simulink model "rlBallandPlate"  (R2023a)
settings: Solver=ode45  StartTime=0.0  StopTime=40  RelTol=1e-3
undefined symbols (not defined in the file): DiscIntNeverNeededParam, Ts
libraries: simulink x3, rllib x1
settings Model: Creator=The MathWorks, Inc.  LastModifiedBy=danieludekwe
settings SolverCC: AlgebraicLoopSolver=TrustRegion  MaxZcPerStep=1
settings DataIOCC: DSMLogging=off  ReturnWorkspaceOutputs=off
settings OptimizationCC: ReuseModelBlockBuffer=off
settings DebuggingCC: UnconnectedInputMsg=warning  UnconnectedOutputMsg=warning  UnconnectedLineMsg=warning
settings HardwareCC: ProdBitPerLong=64  ProdHWDeviceType=Apple->ARM64
settings ModelReferenceCC: EnableRefExpFcnMdlSchedulingChecks=on
settings RTWCC: DLArmComputeVersion=19.05
settings ExplorerConfigSet: InternalSimMechanicsExplorerSettings="<ExplorerConfiguration><canonicalview>default</canonicalview><AnimationSetting><BasePlaybackSpeed>1.0</BasePlaybackSpeed><PlaybackSpeedFactor>1.0</PlaybackSpeedFactor></AnimationSetting><TilePanel><TileInfo><Tiles Columns=\"1\" Count=\"1\" Rows=\"1\"><Column Weight=\"1\"/><Row Weight=\"1\"/><Tile Height=\"1\" Width=\"1\" X=\"0\" Y=\"0\"/></Tiles></TileInfo><SceneInfo><SceneViewer><BGColor><R>1</R><G>1</G><B>1</B></BGColor><Camera><DoPerspective>off</DoPerspective><Position><X>0.835449044511457073</X><Y>-0.495506913595096854</Y><Z>0.970261214764596258</Z></Position><Center><X>0.258098775321831175</X><Y>0.0818433555945289881</Y><Z>0.392910945574970416</Z></Center><Up><X>-0.408248290463863073</X><Y>0.408248290463863073</Y><Z>0.816496580927726145</Z></Up><ViewLimDist>1</ViewLimDist><YLim>0.340419242978096004</YLim><XLim>0.488995507299471222</XLim></Camera></SceneViewer></SceneInfo></TilePanel><MechEditorPanel><Cameras/><GfxPanelCameraMap/><VideoCreator><PlaybackSpeedRatio>1.0</PlaybackSpeedRatio><FrameRate>30</FrameRate><VideoFormat>Motion JPEG AVI</VideoFormat><FrameSize>auto</FrameSize></VideoCreator></MechEditorPanel></ExplorerConfiguration>"

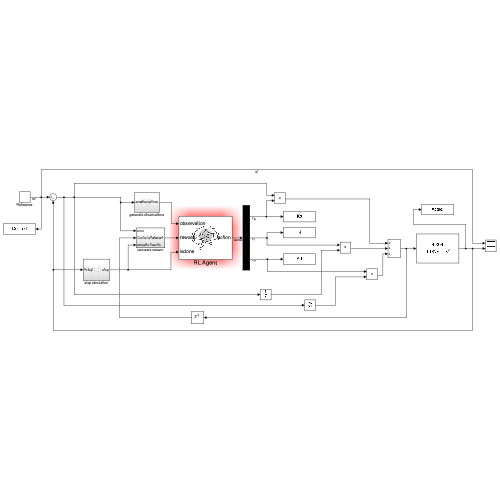
[thumbnail: Simulink's stored preview of the top-level diagram]
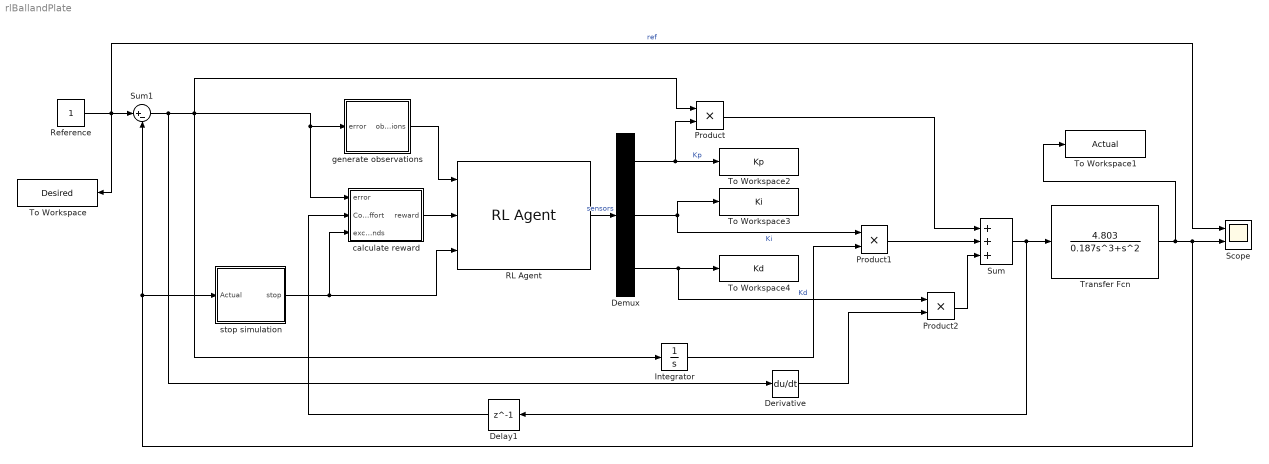
== system rlBallandPlate ==
  Delay1 : Delay  DelayLength=1
  Demux : Demux  Outputs=3
  Derivative : Derivative  CoefficientInTFapproximation=0
  Integrator : Integrator
  Product : Product
  Product1 : Product
  Product2 : Product
  RL Agent : rllib/RL Agent  Agent=agent  ExternalActionAsInput=off  ProvideLastAction=off  ProvideCumRwd=off  TreatAsDirectFeedthrough=on  UseStrictObservationDataTypes=off
  Reference : Constant
  Scope : Scope  NumInputPorts=2
  Sum : Sum  Inputs=+++
  Sum1 : Sum  Inputs=|+-  SaturateOnIntegerOverflow=on
  To Workspace : ToWorkspace  VariableName=Desired  SampleTime=-1
  To Workspace1 : ToWorkspace  VariableName=Actual  SampleTime=-1
  To Workspace2 : ToWorkspace  VariableName=Kp  SaveFormat=Structure With Time  SampleTime=-1
  To Workspace3 : ToWorkspace  VariableName=Ki  SaveFormat=Structure With Time  SampleTime=-1
  To Workspace4 : ToWorkspace  VariableName=Kd  SaveFormat=Structure With Time  SampleTime=-1
  Transfer Fcn : TransferFcn  Numerator=4.803  Denominator=[0.187 1 0 0]
  calculate reward : Subsystem
  generate observations : Subsystem
  stop simulation : Subsystem
  wires:
  generate observations/1(observations) -> RL Agent/1
  stop simulation/1(stop) -> RL Agent/3, calculate reward/3(exceeds bounds)
  Transfer Fcn/1 -> To Workspace1/1, Scope/2, stop simulation/1(Actual), Sum1/2
  RL Agent/1 -> Demux/1  "sensors"
  Reference/1 -> To Workspace/1, Sum1/1, Scope/1  "ref"
  Sum1/1 -> calculate reward/1(error), generate observations/1(error), Integrator/1, Product/1, Derivative/1
  Delay1/1 -> calculate reward/2(Control effort)
  calculate reward/1(reward) -> RL Agent/2
  Demux/2 -> To Workspace3/1, Product1/1  "Ki"
  Demux/3 -> To Workspace4/1, Product2/1  "Kd"
  Product1/1 -> Sum/2
  Product/1 -> Sum/1
  Product2/1 -> Sum/3
  Sum/1 -> Delay1/1, Transfer Fcn/1
  Derivative/1 -> Product2/2
  Integrator/1 -> Product1/2
  Demux/1 -> To Workspace2/1, Product/2  "Kp"

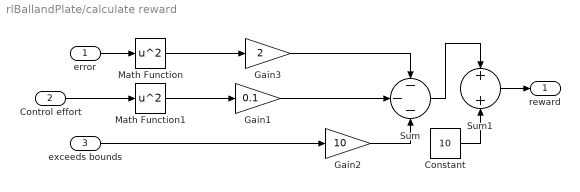
== system rlBallandPlate/calculate reward ==
  error : Inport
  Control effort : Inport  Port=2
  exceeds bounds : Inport  Port=3
  Constant : Constant  Value=10
  Gain1 : Gain  Gain=0.1
  Gain2 : Gain  Gain=10
  Gain3 : Gain  Gain=2
  Math Function : Math  Operator=square
  Math Function1 : Math  Operator=square
  Sum : Sum  Inputs=---  OutDataTypeStr=double
  Sum1 : Sum  OutDataTypeStr=double
  reward : Outport  VectorParamsAs1DForOutWhenUnconnected=off
  wires:
  exceeds bounds/1 -> Gain2/1
  error/1 -> Math Function/1
  Math Function/1 -> Gain3/1
  Gain3/1 -> Sum/1
  Sum/1 -> Sum1/1
  Constant/1 -> Sum1/2
  Sum1/1 -> reward/1
  Math Function1/1 -> Gain1/1
  Gain2/1 -> Sum/3
  Control effort/1 -> Math Function1/1
  Gain1/1 -> Sum/2

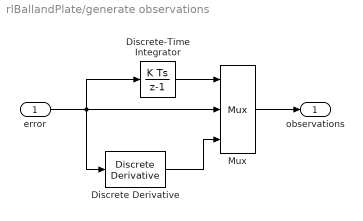
== system rlBallandPlate/generate observations ==
  error : Inport
  Discrete Derivative : simulink/Discrete/Discrete Derivative  gainval=1.0  ICPrevScaledInput=0.0  OutMin=[]  OutMax=[]  OutDataType=fixdt(1, 16)  OutScaling=2^-10  DoSatur=off
  Discrete-Time Integrator : DiscreteIntegrator  SampleTime=Ts  ICPrevOutput=DiscIntNeverNeededParam  ICPrevScaledInput=DiscIntNeverNeededParam
  Mux : Mux  Inputs=3
  observations : Outport  VectorParamsAs1DForOutWhenUnconnected=off
  wires:
  Discrete-Time Integrator/1 -> Mux/1
  Mux/1 -> observations/1
  error/1 -> Discrete Derivative/1, Mux/2, Discrete-Time Integrator/1
  Discrete Derivative/1 -> Mux/3

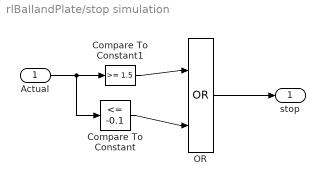
== system rlBallandPlate/stop simulation ==
  Actual : Inport
  Compare To Constant : simulink/Logic and Bit Operations/Compare To Constant  relop=<=  const=-0.1  OutDataTypeStr=boolean
  Compare To Constant1 : simulink/Logic and Bit Operations/Compare To Constant  relop=>=  const=1.5  OutDataTypeStr=boolean
  OR : Logic  Operator=OR  IconShape=distinctive  AllPortsSameDT=off  OutDataTypeStr=boolean
  stop : Outport  VectorParamsAs1DForOutWhenUnconnected=off
  wires:
  Compare To Constant1/1 -> OR/1
  Actual/1 -> Compare To Constant/1, Compare To Constant1/1
  Compare To Constant/1 -> OR/2
  OR/1 -> stop/1
